simulink model "dashboard_light"  (R2020b)
settings: Solver=VariableStepAuto  StartTime=0.0  StopTime=10  RelTol=1e-3
settings Model: Creator=Training  LastModifiedBy=Training

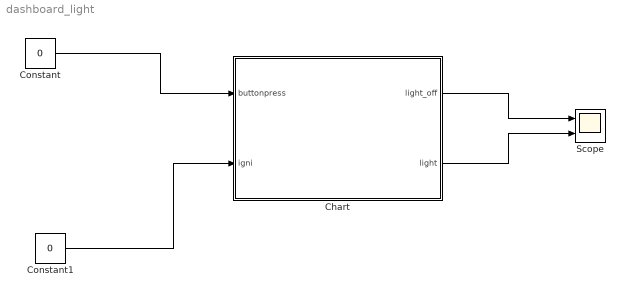
== system dashboard_light ==
  Chart : Stateflow chart  TreatAsAtomicUnit=on
  Constant : Constant  Value=0
  Constant1 : Constant  Value=0
  Scope : Scope  NumInputPorts=2
  wires:
  Chart/1(light_off) -> Scope/1
  Constant1/1 -> Chart/2(igni)
  Constant/1 -> Chart/1(buttonpress)
  Chart/2(light) -> Scope/2

== stateflow chart dashboard_light/Chart ==
  state DBlightoff
    entry:
    sysstate=2;
    light_off=~light;
  state DBlighton
    entry :
    sysstate=1;
    light=1;
  (default) -> DBlighton : {light==0;}
  DBlighton -> DBlightoff : [igni==1 && buttonpress==0]
  DBlightoff -> DBlighton : [igni==1||buttonpress==1]
  data: buttonpress input; igni input; light_off output; sysstate local; light output
